simulink model "testflightconditions"  (R2012b)
settings: Solver=ode45  StartTime=0.0  StopTime=10.0  RelTol=1e-3
libraries: simulink x1
settings Model: Creator=tlavelle  LastModifiedBy=tlavelle

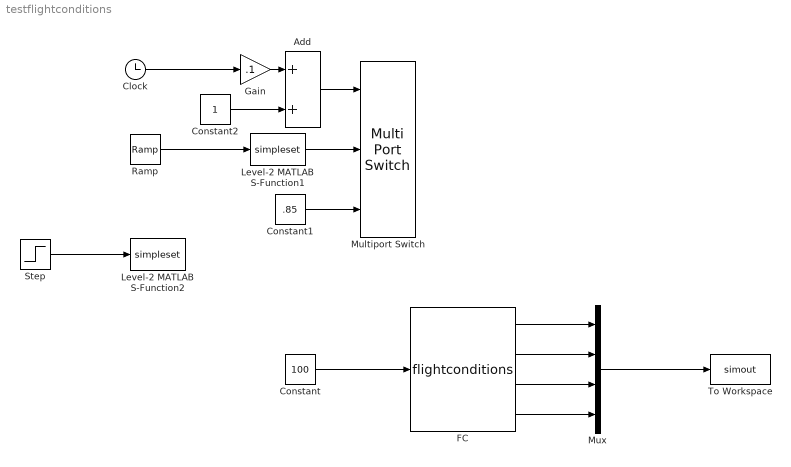
== system testflightconditions ==
  Add : Sum
  Clock : Clock
  Constant : Constant  Value=100
  Constant1 : Constant  Value=.85
  Constant2 : Constant
  FC : M-S-Function  FunctionName=flightconditions  Parameters=alt,MN,dTs  mask{alt=100000, MN=0.85, dTs=0}
      mask prompts: alt "altitude"; MN "Mach Number"; dTs "Ambient Temperature Delta"
      mask Display:
      | color('blue'); port_label('input',1,'Weight Flow')
      | 
      | color('red'); port_label('output',1,'Flow Out')
      | color('red'); port_label('output',2,'Ambient Pressure')
      | color('green'); port_label('output',3,'Fram')
  Gain : Gain  Gain=.1
  Level-2 MATLAB S-Function1 : M-S-Function  FunctionName=simpleset  Parameters='alt'
  Level-2 MATLAB S-Function2 : M-S-Function  FunctionName=simpleset  Parameters='MN'
  Multiport Switch : MultiPortSwitch  Inputs=2
  Mux : Mux
  Ramp : simulink/Sources/Ramp  slope=10000  start=0  X0=0
  Step : Step  Time=10  After=.85  SampleTime=0
  To Workspace : ToWorkspace  VariableName=simout  SampleTime=-1  SaveFormat=Timeseries
  wires:
  Constant/1 -> FC/1
  Ramp/1 -> Level-2 MATLAB S-Function1/1
  Step/1 -> Level-2 MATLAB S-Function2/1
  Level-2 MATLAB S-Function1/1 -> Multiport Switch/2
  Constant1/1 -> Multiport Switch/3
  Clock/1 -> Gain/1
  Gain/1 -> Add/1
  Add/1 -> Multiport Switch/1
  Constant2/1 -> Add/2
  Mux/1 -> To Workspace/1
  FC/1 -> Mux/1
  FC/2 -> Mux/2
  FC/3 -> Mux/3
  FC/4 -> Mux/4
